simulink model "Improved_IMC_structure"  (R2017b)
settings: Solver=ode3  StartTime=0.0  StopTime=Ttotal*10  FixedStep=Tsample  RelTol=1e-3
values from neighbouring files (symbols this model uses):
  capacitor = 470e-6    (= 0.00047)    [Improved_IMC_structure_input.m]
  dutyCycle = 1-inputVoltage/outputVoltage    (= 0.5)    [Improved_IMC_structure_input.m]
  inductor = 833e-3    (= 0.833)    [Improved_IMC_structure_input.m]
  Kd_proposed = Kp_proposed*Td_proposed    [Improved_IMC_structure_input.m]
  Ki_proposed = Kp_proposed/Ti_proposed    [Improved_IMC_structure_input.m]
  Kp_proposed = 2*undampedNaturalFreq*dampingRatio/(openLoopGain*timeconst)    [Improved_IMC_structure_input.m]
  openLoopGain = inputVoltage/inductor/capacitor    (= 15325.2790478)    [Improved_IMC_structure_input.m]
  openLoopZero = -inductorCurrent*inductor/inputVoltage    (= -0.3332)    [Improved_IMC_structure_input.m]
  resistor = 10    [Improved_IMC_structure_input.m]
  Vo = outputVoltage    (= 12)    [Improved_IMC_structure_input.m]    (also in plot_improved_IMC_control.m = ScopeData1.signals(4).values; plot_result.m = ScopeData1.signals(4).values)
libraries: simulink x1
settings Model: Creator=liush  LastModifiedBy=liush

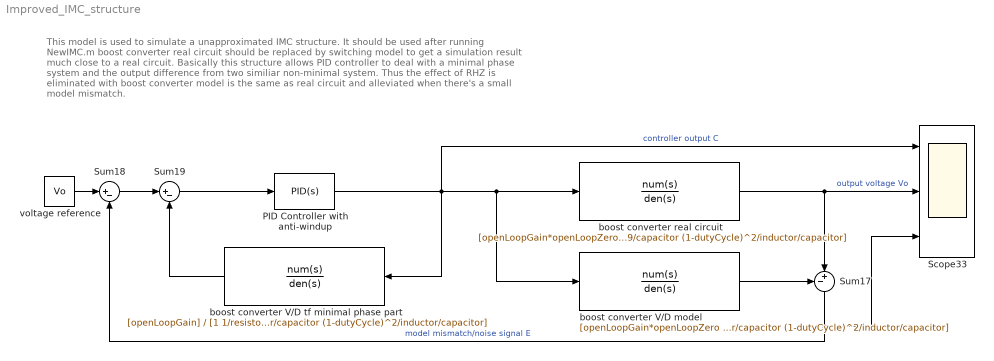
== system Improved_IMC_structure ==
  note: This model is used to simulate a unapproximated IMC structure.
      | It should be used after running NewIMC.m
      | boost converter real circuit should be replaced by switching model to get a simulation result much close to a real circuit.
      | Basically this structure allows PID controller to deal with a minimal phase system and the output difference from two similiar
      | non-minimal system. Thus the effect of RHZ is eliminated with boost converter model is the same as real circuit and alleviated
      | when there's a small model mismatch.
  PID Controller with anti-windup : simulink/Continuous/PID Controller  Controller=PID  TimeDomain=Continuous-time  SampleTime=-1  IntegratorMethod=Forward Euler  FilterMethod=Forward Euler  Form=Parallel  UseFilter=on  ControllerParametersSource=internal  P=Kp_proposed  I=Ki_proposed  D=Kd_proposed  N=10000  InitialConditionSource=internal  InitialConditionForIntegrator=0  InitialConditionForFilter=0  ExternalReset=none  LimitOutput=on  UpperSaturationLimit=1  LowerSaturationLimit=0  LinearizeAsGain=on  AntiWindupMode=clamping  Kb=1  TrackingMode=off  Kt=1  PParamMin=[]  PParamMax=[]  IParamMin=[]  IParamMax=[]  DParamMin=[]  DParamMax=[]  NParamMin=[]  NParamMax=[]  KbParamMin=[]  KbParamMax=[]  KtParamMin=[]  KtParamMax=[]  POutMin=[]  POutMax=[]  IOutMin=[]  IOutMax=[]  DOutMin=[]  DOutMax=[]  NOutMin=[]  NOutMax=[]  KbOutMin=[]  KbOutMax=[]  KtOutMin=[]  KtOutMax=[]  IntegratorOutMin=[]  IntegratorOutMax=[]  FilterOutMin=[]  FilterOutMax=[]  SumOutMin=[]  SumOutMax=[]  SumI1OutMin=[]  SumI1OutMax=[]  SumI2OutMin=[]  SumI2OutMax=[]  SumI3OutMin=[]  SumI3OutMax=[]  SumDOutMin=[]  SumDOutMax=[]  SaturationOutMin=[]  SaturationOutMax=[]  IntegratorContinuousStateAttributes=''  IntegratorStateMustResolveToSignalObject=off  IntegratorRTWStateStorageClass=Auto  FilterContinuousStateAttributes=''  FilterStateMustResolveToSignalObject=off  FilterRTWStateStorageClass=Auto  DifferentiatorICPrevScaledInput=0  DifferentiatorOutMin=[]  DifferentiatorOutMax=[]  InitialConditionSetting=State (most efficient)  FilterDiffOutCoefMin=[]  FilterDiffOutCoefMax=[]  SumDenOutMin=[]  SumDenOutMax=[]  SumNumOutMin=[]  SumNumOutMax=[]  ReciprocalOutMin=[]  ReciprocalOutMax=[]  DivideOutMin=[]  DivideOutMax=[]  TunerSelectOption=Transfer Function Based (PID Tuner App)
  Scope33 : Scope  NumInputPorts=3
  Sum17 : Sum  Inputs=-+|
  Sum18 : Sum  Inputs=|+-
  Sum19 : Sum  Inputs=|+-
  boost converter V/D model : TransferFcn  Numerator=[openLoopGain*openLoopZero openLoopGain]  Denominator=[1 1/resistor/capacitor (1-dutyCycle)^2/inductor/capacitor]
  boost converter V/D tf minimal phase part : TransferFcn  Numerator=[openLoopGain]  Denominator=[1 1/resistor/capacitor (1-dutyCycle)^2/inductor/capacitor]
  boost converter real circuit : TransferFcn  Numerator=[openLoopGain*openLoopZero openLoopGain]  Denominator=[1 1/resistor*0.9/capacitor (1-dutyCycle)^2/inductor/capacitor]
  voltage reference : Constant  Value=Vo
  wires:
  Sum18/1 -> Sum19/1
  Sum19/1 -> PID Controller with anti-windup/1
  Sum17/1 -> Scope33/3, Sum18/2  "model mismatch/noise signal E"
  voltage reference/1 -> Sum18/1
  boost converter real circuit/1 -> Scope33/2, Sum17/2  "output voltage Vo"
  PID Controller with anti-windup/1 -> Scope33/1, boost converter V/D tf minimal phase part/1, boost converter real circuit/1, boost converter V/D model/1  "controller output C"
  boost converter V/D model/1 -> Sum17/1
  boost converter V/D tf minimal phase part/1 -> Sum19/2
